simulink subsystem "SimpleEngine"  (R2024b)
settings: Solver=VariableStepAuto  StartTime=0.0  StopTime=10.0  RelTol=1e-3
undefined symbols (not defined in the file): Afr, BSFC, CrkAng, EngSpdOut, EngTrq, ExhManGasTemp, FuelFlw, FuelVolFlw, IntkPortFlw, NormAirChrg, PlntEngTimeCECP, PlntEngTimeCEGR, PlntEngTimeCETC, PlntEngTimeCICP, PlntEngTimeCIRL, PlntEngTimeCIVL, PlntEngTimeCVCR, PlntEngTimeCVGT, PlntEngTimeCWGA, PlntEngTimeCWVA
libraries: autolibsharedcommon x1, autolibpowerinfoutils x1, autolibsharedmappedengines x1, autolibutils x1
settings Model: ModifiedByFormat=The MathWorks, Inc.  Creator=The MathWorks, Inc.  LastModifiedBy=The MathWorks, Inc.
settings SolverCC: MaxZcPerStep=1
settings OptimizationCC: ReuseModelBlockBuffer=off
settings DebuggingCC: UnconnectedInputMsg=warning  UnconnectedOutputMsg=warning  UnconnectedLineMsg=warning
settings ModelReferenceCC: EnableRefExpFcnMdlSchedulingChecks=on
settings RTWCC: GPUComputeCapability=3.5  DLArmComputeVersion=19.05

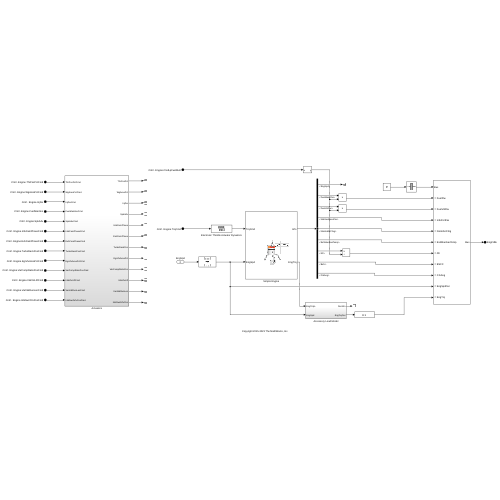
[thumbnail: Simulink's stored preview of the top-level diagram]
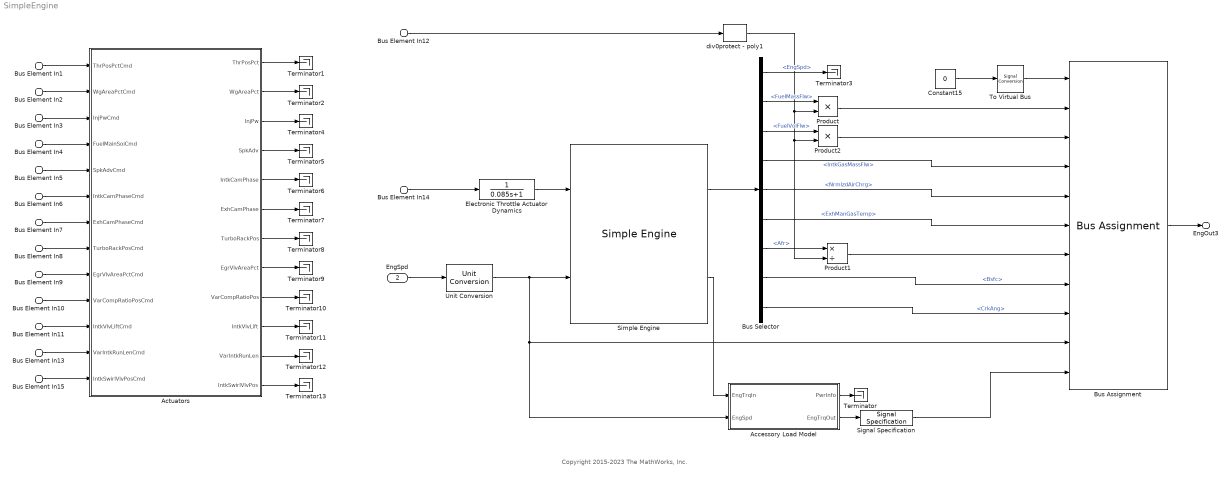
== system SimpleEngine ==
  note: Copyright 2015-2023 The MathWorks, Inc.
  Bus Element In12 : Inport  PortName=Cntrl  Element=Engine.ClsdLpFuelMult
  Bus Element In14 : Inport  PortName=Cntrl  Element=Engine.TrqCmd
  Bus Element In1 : Inport  PortName=Cntrl  Element=Engine.ThrPosPctCmd
  Bus Element In2 : Inport  PortName=Cntrl  Element=Engine.WgAreaPctCmd
  Bus Element In3 : Inport  PortName=Cntrl  Element=Engine.InjPw
  Bus Element In4 : Inport  PortName=Cntrl  Element=Engine.FuelMainSoi
  Bus Element In5 : Inport  PortName=Cntrl  Element=Engine.SpkAdv
  Bus Element In6 : Inport  PortName=Cntrl  Element=Engine.IntkCamPhaseCmd
  Bus Element In7 : Inport  PortName=Cntrl  Element=Engine.ExhCamPhaseCmd
  Bus Element In8 : Inport  PortName=Cntrl  Element=Engine.TurboRackPosCmd
  Bus Element In9 : Inport  PortName=Cntrl  Element=Engine.EgrVlvAreaPctCmd
  Bus Element In10 : Inport  PortName=Cntrl  Element=Engine.VarCompRatioPosCmd
  Bus Element In11 : Inport  PortName=Cntrl  Element=Engine.IntkVlvLiftCmd
  Bus Element In13 : Inport  PortName=Cntrl  Element=Engine.VarIntkRunLenCmd
  Bus Element In15 : Inport  PortName=Cntrl  Element=Engine.IntkSwirlVlvPosCmd
  EngSpd : Inport  Port=2  Unit=rad/sec
  Accessory Load Model : Subsystem
  Actuators : Subsystem
  Bus Assignment : BusAssignment  AssignedSignals=FuelFlw,FuelVolFlw,IntkPortFlw,NormAirChrg,ExhManGasTemp,Afr,BSFC,CrkAng,EngSpdOut,EngTrq
  Bus Selector : BusSelector  OutputSignals=EngSpd,FuelMassFlw,FuelVolFlw,IntkGasMassFlw,NrmlzdAirChrg,ExhManGasTemp,Afr,Bsfc,CrkAng
  Constant15 : Constant  Value=0  OutDataTypeStr=Bus: EngineBUS  SampleTime=Inf
  Electronic Throttle Actuator Dynamics : TransferFcn  Denominator=[0.085 1]
  Product : Product
  Product1 : Product  Inputs=*/
  Product2 : Product
  Signal Specification : SignalSpecification  Dimensions=1
  Simple Engine : autolibsharedmappedengines/Simple Engine  f_tqmax=PlntEngTqMax  f_tqmax_n_bpt=PlntEngTqMaxBpt  Lhv=PlntEngFuelLhv  Sg=PlntEngFuelSg  BsfcAvg=PlntEngBsfcAvg  aMode=6
  Terminator{,1..13} (14 alike) : Terminator
  To Virtual Bus : SignalConversion  ConversionOutput=Virtual bus  OverrideOpt=off
  Unit Conversion : UnitConversion
  div0protect - poly1 : autolibutils/div0protect - poly  thresh=0.01  ZeroCross1=off  aMode=6
  EngOut3 : Outport  PortName=EngFdbk
  wires:
  Actuators/12(IntkSwirlVlvPos) -> Terminator13/1
  Actuators/11(VarIntkRunLen) -> Terminator12/1
  Actuators/10(IntkVlvLift) -> Terminator11/1
  Actuators/9(VarCompRatioPos) -> Terminator10/1
  Actuators/8(EgrVlvAreaPct) -> Terminator9/1
  Actuators/7(TurboRackPos) -> Terminator8/1
  Actuators/6(ExhCamPhase) -> Terminator7/1
  Actuators/5(IntkCamPhase) -> Terminator6/1
  Actuators/4(SpkAdv) -> Terminator5/1
  Actuators/3(InjPw) -> Terminator4/1
  Actuators/2(WgAreaPct) -> Terminator2/1
  Actuators/1(ThrPosPct) -> Terminator1/1
  Bus Element In8/1 -> Actuators/8(TurboRackPosCmd)
  Bus Element In15/1 -> Actuators/13(IntkSwirlVlvPosCmd)
  Bus Element In11/1 -> Actuators/11(IntkVlvLiftCmd)
  Bus Element In2/1 -> Actuators/2(WgAreaPctCmd)
  Bus Element In10/1 -> Actuators/10(VarCompRatioPosCmd)
  Bus Element In7/1 -> Actuators/7(ExhCamPhaseCmd)
  Bus Element In5/1 -> Actuators/5(SpkAdvCmd)
  Bus Element In6/1 -> Actuators/6(IntkCamPhaseCmd)
  Bus Element In1/1 -> Actuators/1(ThrPosPctCmd)
  Bus Element In3/1 -> Actuators/3(InjPwCmd)
  Bus Element In4/1 -> Actuators/4(FuelMainSoiCmd)
  Bus Element In9/1 -> Actuators/9(EgrVlvAreaPctCmd)
  Bus Element In13/1 -> Actuators/12(VarIntkRunLenCmd)
  Bus Assignment/1 -> EngOut3/1
  Constant15/1 -> To Virtual Bus/1
  To Virtual Bus/1 -> Bus Assignment/1
  Signal Specification/1 -> Bus Assignment/11
  Unit Conversion/1 -> Simple Engine/2, Bus Assignment/10, Accessory Load Model/2(EngSpd)
  Bus Selector/8 -> Bus Assignment/8  "<Bsfc>"
  Simple Engine/1 -> Bus Selector/1
  Product2/1 -> Bus Assignment/3
  Electronic Throttle Actuator Dynamics/1 -> Simple Engine/1
  Bus Selector/2 -> Product/1  "<FuelMassFlw>"
  Bus Selector/7 -> Product1/1  "<Afr>"
  Bus Selector/4 -> Bus Assignment/4  "<IntkGasMassFlw>"
  Product1/1 -> Bus Assignment/7
  Bus Element In14/1 -> Electronic Throttle Actuator Dynamics/1
  Bus Selector/3 -> Product2/1  "<FuelVolFlw>"
  Accessory Load Model/1(PwrInfo) -> Terminator/1
  div0protect - poly1/1 -> Product2/2, Product1/2, Product/2
  Bus Selector/5 -> Bus Assignment/5  "<NrmlzdAirChrg>"
  Accessory Load Model/2(EngTrqOut) -> Signal Specification/1
  EngSpd/1 -> Unit Conversion/1
  Bus Element In12/1 -> div0protect - poly1/1
  Bus Selector/6 -> Bus Assignment/6  "<ExhManGasTemp>"
  Product/1 -> Bus Assignment/2
  Bus Selector/1 -> Terminator3/1  "<EngSpd>"
  Bus Selector/9 -> Bus Assignment/9  "<CrkAng>"
  Simple Engine/2 -> Accessory Load Model/1(EngTrqIn)

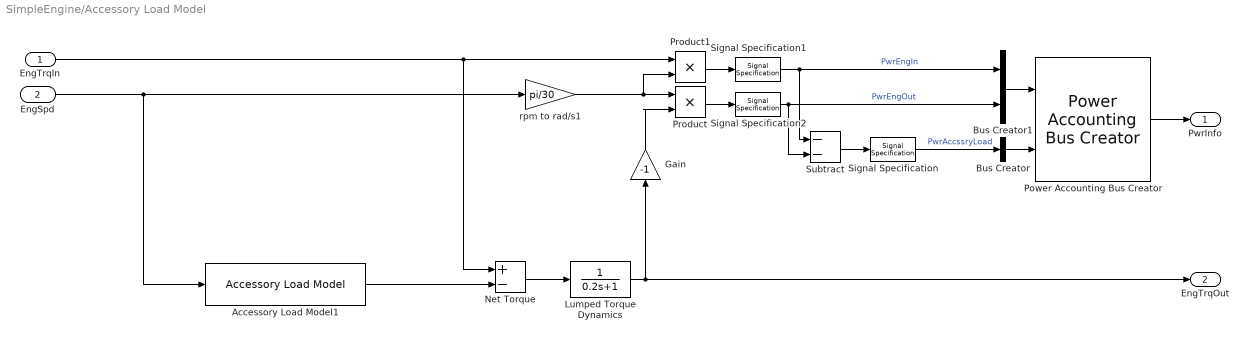
== system SimpleEngine/Accessory Load Model ==
  EngTrqIn : Inport
  EngSpd : Inport  Port=2
  Accessory Load Model1 : autolibsharedcommon/Accessory Load Model  AccPwrTbl=PlntEngAccPwrTbl  AccSpdBpts=PlntEngAccSpdBpt  aMode=aMode
  Bus Creator : BusCreator  Inputs=1
  Bus Creator1 : BusCreator  Inputs=2
  Gain : Gain  Gain=-1
  Lumped Torque Dynamics : TransferFcn  Denominator=[0.2 1]
  Net Torque : Sum  Inputs=+-
  Power Accounting Bus Creator : autolibpowerinfoutils/Power Accounting Bus Creator  AssctBlkSelPopup=Parent  RefBlkName='libraryname/blkname'  PwrTrnsfrdCheckBox=on  PwrNotTrnsfrdCheckBox=on  PwrStoredCheckBox=off  aMode=6
  Product : Product
  Product1 : Product
  Signal Specification : SignalSpecification  Unit=W
  Signal Specification1 : SignalSpecification  Unit=W
  Signal Specification2 : SignalSpecification  Unit=W
  Subtract : Sum  Inputs=--
  rpm to rad/s1 : Gain  Gain=pi/30
  PwrInfo : Outport  VectorParamsAs1DForOutWhenUnconnected=off
  EngTrqOut : Outport  Port=2  Unit=N*m  VectorParamsAs1DForOutWhenUnconnected=off
  wires:
  Accessory Load Model1/1 -> Net Torque/2
  EngSpd/1 -> rpm to rad/s1/1, Accessory Load Model1/1
  Lumped Torque Dynamics/1 -> EngTrqOut/1, Gain/1
  Net Torque/1 -> Lumped Torque Dynamics/1
  Bus Creator/1 -> Power Accounting Bus Creator/2
  Bus Creator1/1 -> Power Accounting Bus Creator/1
  EngTrqIn/1 -> Product1/1, Net Torque/1
  Subtract/1 -> Signal Specification/1
  Signal Specification/1 -> Bus Creator/1  "PwrAccssryLoad"
  Power Accounting Bus Creator/1 -> PwrInfo/1
  Product/1 -> Signal Specification2/1
  Product1/1 -> Signal Specification1/1
  rpm to rad/s1/1 -> Product1/2, Product/1
  Signal Specification1/1 -> Subtract/1, Bus Creator1/1  "PwrEngIn"
  Signal Specification2/1 -> Subtract/2, Bus Creator1/2  "PwrEngOut"
  Gain/1 -> Product/2

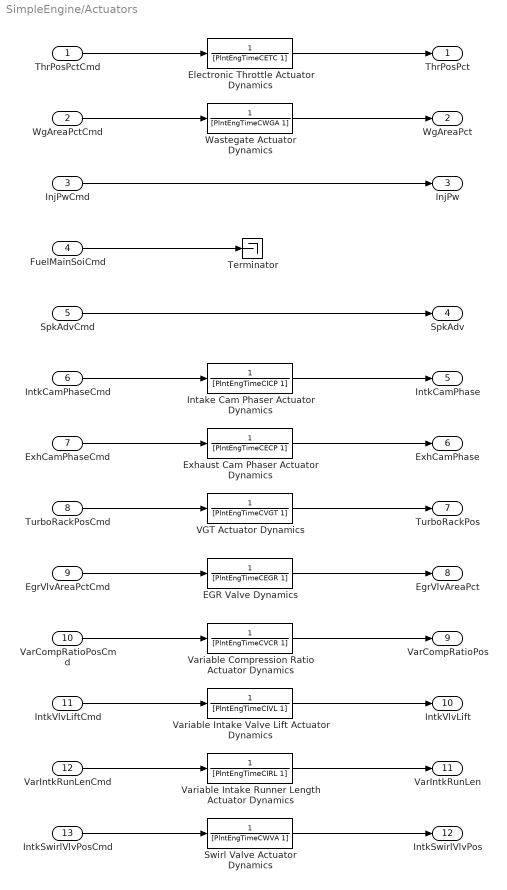
== system SimpleEngine/Actuators ==
  ThrPosPctCmd : Inport  Unit=%
  WgAreaPctCmd : Inport  Port=2  Unit=%
  InjPwCmd : Inport  Port=3  Unit=ms
  FuelMainSoiCmd : Inport  Port=4  Unit=deg
  SpkAdvCmd : Inport  Port=5  Unit=deg
  IntkCamPhaseCmd : Inport  Port=6  Unit=deg
  ExhCamPhaseCmd : Inport  Port=7  Unit=deg
  TurboRackPosCmd : Inport  Port=8  Unit=1
  EgrVlvAreaPctCmd : Inport  Port=9  Unit=%
  VarCompRatioPosCmd : Inport  Port=10
  IntkVlvLiftCmd : Inport  Port=11
  VarIntkRunLenCmd : Inport  Port=12
  IntkSwirlVlvPosCmd : Inport  Port=13
  EGR Valve Dynamics : TransferFcn  Denominator=[PlntEngTimeCEGR 1]
  Electronic Throttle Actuator Dynamics : TransferFcn  Denominator=[PlntEngTimeCETC 1]
  Exhaust Cam Phaser Actuator Dynamics : TransferFcn  Denominator=[PlntEngTimeCECP 1]
  Intake Cam Phaser Actuator Dynamics : TransferFcn  Denominator=[PlntEngTimeCICP 1]
  Swirl Valve Actuator Dynamics : TransferFcn  Denominator=[PlntEngTimeCWVA 1]
  Terminator : Terminator
  VGT Actuator Dynamics : TransferFcn  Denominator=[PlntEngTimeCVGT 1]
  Variable Compression Ratio Actuator Dynamics : TransferFcn  Denominator=[PlntEngTimeCVCR 1]
  Variable Intake Runner Length Actuator Dynamics : TransferFcn  Denominator=[PlntEngTimeCIRL 1]
  Variable Intake Valve Lift Actuator Dynamics : TransferFcn  Denominator=[PlntEngTimeCIVL 1]
  Wastegate Actuator Dynamics : TransferFcn  Denominator=[PlntEngTimeCWGA 1]
  ThrPosPct : Outport  Unit=%  VectorParamsAs1DForOutWhenUnconnected=off
  WgAreaPct : Outport  Port=2  Unit=%  VectorParamsAs1DForOutWhenUnconnected=off
  InjPw : Outport  Port=3  VectorParamsAs1DForOutWhenUnconnected=off
  SpkAdv : Outport  Port=4  VectorParamsAs1DForOutWhenUnconnected=off
  IntkCamPhase : Outport  Port=5  Unit=deg  VectorParamsAs1DForOutWhenUnconnected=off
  ExhCamPhase : Outport  Port=6  Unit=deg  VectorParamsAs1DForOutWhenUnconnected=off
  TurboRackPos : Outport  Port=7  Unit=1  VectorParamsAs1DForOutWhenUnconnected=off
  EgrVlvAreaPct : Outport  Port=8  Unit=%  VectorParamsAs1DForOutWhenUnconnected=off
  VarCompRatioPos : Outport  Port=9  VectorParamsAs1DForOutWhenUnconnected=off
  IntkVlvLift : Outport  Port=10  VectorParamsAs1DForOutWhenUnconnected=off
  VarIntkRunLen : Outport  Port=11  VectorParamsAs1DForOutWhenUnconnected=off
  IntkSwirlVlvPos : Outport  Port=12  VectorParamsAs1DForOutWhenUnconnected=off
  wires:
  Variable Compression Ratio Actuator Dynamics/1 -> VarCompRatioPos/1
  Variable Intake Valve Lift Actuator Dynamics/1 -> IntkVlvLift/1
  Variable Intake Runner Length Actuator Dynamics/1 -> VarIntkRunLen/1
  Swirl Valve Actuator Dynamics/1 -> IntkSwirlVlvPos/1
  Intake Cam Phaser Actuator Dynamics/1 -> IntkCamPhase/1
  Exhaust Cam Phaser Actuator Dynamics/1 -> ExhCamPhase/1
  Wastegate Actuator Dynamics/1 -> WgAreaPct/1
  Electronic Throttle Actuator Dynamics/1 -> ThrPosPct/1
  FuelMainSoiCmd/1 -> Terminator/1
  IntkVlvLiftCmd/1 -> Variable Intake Valve Lift Actuator Dynamics/1
  IntkSwirlVlvPosCmd/1 -> Swirl Valve Actuator Dynamics/1
  WgAreaPctCmd/1 -> Wastegate Actuator Dynamics/1
  ThrPosPctCmd/1 -> Electronic Throttle Actuator Dynamics/1
  ExhCamPhaseCmd/1 -> Exhaust Cam Phaser Actuator Dynamics/1
  IntkCamPhaseCmd/1 -> Intake Cam Phaser Actuator Dynamics/1
  VarCompRatioPosCmd/1 -> Variable Compression Ratio Actuator Dynamics/1
  VarIntkRunLenCmd/1 -> Variable Intake Runner Length Actuator Dynamics/1
  InjPwCmd/1 -> InjPw/1
  VGT Actuator Dynamics/1 -> TurboRackPos/1
  EGR Valve Dynamics/1 -> EgrVlvAreaPct/1
  TurboRackPosCmd/1 -> VGT Actuator Dynamics/1
  EgrVlvAreaPctCmd/1 -> EGR Valve Dynamics/1
  SpkAdvCmd/1 -> SpkAdv/1
